simulink model "MainSwitch"  (R2017b)
settings: Solver=VariableStepAuto  StartTime=0.0  StopTime=10.0  RelTol=1e-3
settings Model: Creator=segadiallo  LastModifiedBy=segadiallo

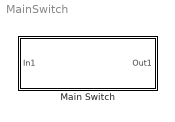
== system MainSwitch ==
  Main Switch : Subsystem
      mask help: Main Switch
      mask Display:
      | disp('Main Switch')
      | port_label('output',1,'inputV')
      | port_label('input',1,'Go')

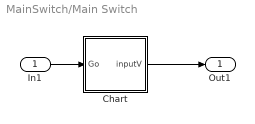
== system MainSwitch/Main Switch ==
  In1 : Inport
  Chart : Stateflow chart  TreatAsAtomicUnit=on
  Out1 : Outport
  wires:
  Chart/1(inputV) -> Out1/1
  In1/1 -> Chart/1(Go)

== stateflow chart MainSwitch/Main Switch/Chart ==
  state START
    entry:
    y=0
  state CONNECT
    entry: tcpInit;
  state DISCONNECT
    entry: y=0
    coder.extrinsic('evalin')
    obj=evalin('base','objWs')
    fclose(obj)
  state Toggle
    entry: y = y + 1
    if y==3
    y=1
    end
  state SerialControl1
    entry: y==1
  (default) -> START
  START -> CONNECT : [n==1]
  DISCONNECT -> CONNECT : [n==1]
  CONNECT -> DISCONNECT [order 1] : [n==0]
  SerialControl1 -> DISCONNECT [order 2] : [n==0]
  CONNECT -> SerialControl1 [order 2]
  Toggle -> SerialControl1 : after(1,sec)
  SerialControl1 -> Toggle [order 1] : [n==1]
  data: Go input; inputV output
  function tcpInit:
    | function tcpInit
    | coder.extrinsic('tcpip');
    | coder.extrinsic('assignin');
    | persistent obj
    | if isempty(obj)
    |     obj=tcpip('10.0.0.1',9001);
    |     assignin('base','objWs',obj);
    |  
    |     set(obj,'Terminator','LF');
    | set(obj,'InputBufferSize',1000)
    | set(obj, 'Timeout', .5)
    | set(obj, 'ByteOrder','bigEndian');
    | 
    |  
    |  fopen(obj);
    |  
    |  fwrite(obj,128);
    | pause(.1)
    | 
    | fwrite(obj,132);
    | pause(.1)
    | 
    | % %Print 'go' on display
    | fwrite(obj, [164, 71, 79, 32, 32]);
    | % make a sound
    | fwrite(obj, [140 1 3 60 20 72 20 84 40 ]); %RoombaInit Song
    | fwrite(obj, [140 2 1 60 20]); % BeepRoomba song
    | fwrite(obj, [140 3 3 84 20 72 30 60 40]); % PowerOffRoomba song
    | fwrite(obj, [141 1]); % play RoombaInit song
    | pause(1);
    | so=obj;
    | end
